simulink model "simplePos"  (R2016b)
settings: Solver=VariableStepAuto  StartTime=0.0  StopTime=100.0  RelTol=1e-3
settings Model: Creator=Roozbeh  LastModifiedBy=Roozbeh

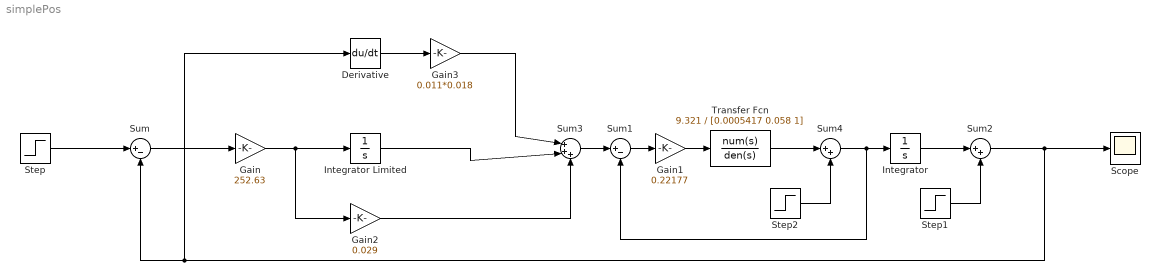
== system simplePos ==
  Derivative : Derivative
  Gain : Gain  Gain=252.63
  Gain1 : Gain  Gain=0.22177
  Gain2 : Gain  Gain=0.029
  Gain3 : Gain  Gain=0.011*0.018
  Integrator : Integrator
  Integrator Limited : Integrator  LimitOutput=on  UpperSaturationLimit=1  LowerSaturationLimit=0
  Scope : Scope
  Step : Step  SampleTime=0
  Step1 : Step  Time=10  After=2  SampleTime=0
  Step2 : Step  Time=10  After=2  SampleTime=0
  Sum : Sum  Inputs=|+-
  Sum1 : Sum  Inputs=|+-
  Sum2 : Sum  Inputs=|++
  Sum3 : Sum  Inputs=|+++
  Sum4 : Sum  Inputs=|++
  Transfer Fcn : TransferFcn  Numerator=9.321  Denominator=[0.0005417 0.058 1]
  wires:
  Sum/1 -> Gain/1
  Step/1 -> Sum/1
  Sum1/1 -> Gain1/1
  Gain1/1 -> Transfer Fcn/1
  Gain/1 -> Integrator Limited/1, Gain2/1
  Derivative/1 -> Gain3/1
  Gain2/1 -> Sum3/3
  Integrator Limited/1 -> Sum3/2
  Gain3/1 -> Sum3/1
  Sum2/1 -> Derivative/1, Sum/2, Scope/1
  Integrator/1 -> Sum2/1
  Step1/1 -> Sum2/2
  Sum3/1 -> Sum1/1
  Sum4/1 -> Sum1/2, Integrator/1
  Transfer Fcn/1 -> Sum4/1
  Step2/1 -> Sum4/2
